simulink model "clothoidSequenceSimulation"  (R2022a)
settings: Solver=ode45  StartTime=0.0  StopTime=S  MaxStep=.1  RelTol=1e-3  EnableMultiTasking=on
values from neighbouring files (symbols this model uses):
  theta0 = 5/180*pi    (= 0.0872664625997)    [errorConnection_v1.m]    (also in errorConnection_v2.m; errorConnection_v3.m = 0.174532925199)
  y0 = 0.5    [errorConnection_v2.m]    (also in errorConnection_v3.m = 0)
settings Model: Creator=klaus  LastModifiedBy=schmidt
settings SolverCC: AlgebraicLoopSolver=TrustRegion
settings DataIOCC: LimitDataPoints=on  SaveFormat=Array  ReturnWorkspaceOutputs=off
settings OptimizationCC: LifeSpan=inf
settings DebuggingCC: UnderspecifiedInitializationDetection=Classic  MergeDetectMultiDrivingBlocksExec=none  SolverPrmCheckMsg=warning  UnconnectedInputMsg=warning  UnconnectedOutputMsg=warning  UnconnectedLineMsg=warning  StateNameClashWarn=warning  SFUnexpectedBacktrackingDiag=warning  SFNoUnconditionalDefaultTransitionDiag=warning  SFExecutionAtInitializationDiag=none  SFMachineParentedDataDiag=warning  ArithmeticOperatorsInVariantConditions=warning
settings HardwareCC: ProdBitPerPointer=32  ProdBitPerSizeT=32  ProdBitPerPtrDiffT=32  ProdLargestAtomicFloat=None  ProdIntDivRoundTo=Undefined  ProdEndianess=Unspecified  ProdWordSize=32  ProdHWDeviceType=32-bit Generic
settings ModelReferenceCC: PropagateSignalLabelsOutOfModel=off
settings SFSimCC: SimUseLocalCustomCode=off  CustomCodeUndefinedFunction=UseInterfaceOnly
settings RTWCC: RTWUseLocalCustomCode=off
settings CodeAppCC: StateflowObjectComments=on
settings GRTTargetCC: TargetLangStandard=C89/C90 (ANSI)
settings ConfigComp: CovMetricSettings=dw  CovSaveCumulativeToWorkspaceVar=on  CovSaveSingleToWorkspaceVar=on  CovExternalEMLEnable=off

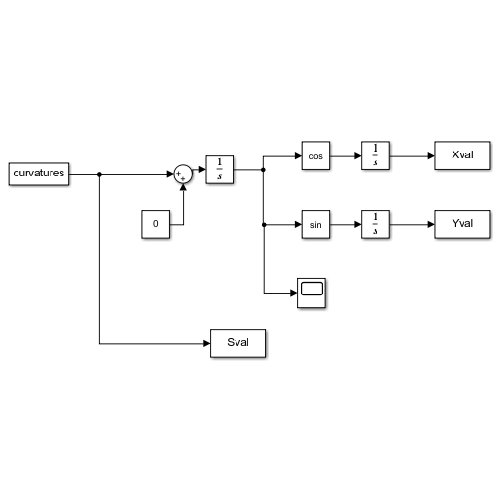
[thumbnail: Simulink's stored preview of the top-level diagram]
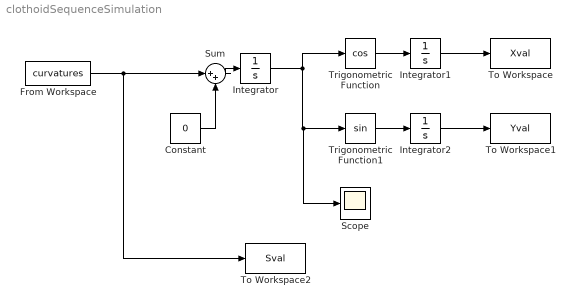
== system clothoidSequenceSimulation ==
  Constant : Constant  Value=0
  From Workspace : FromWorkspace  VariableName=curvatures
  Integrator : Integrator  InitialCondition=theta0
  Integrator1 : Integrator
  Integrator2 : Integrator  InitialCondition=y0
  Scope : Scope
  Sum : Sum  Inputs=|++
  To Workspace : ToWorkspace  VariableName=Xval  SampleTime=-1
  To Workspace1 : ToWorkspace  VariableName=Yval  SampleTime=-1
  To Workspace2 : ToWorkspace  VariableName=Sval  SampleTime=-1
  Trigonometric Function : Trigonometry  Operator=cos
  Trigonometric Function1 : Trigonometry
  wires:
  Integrator/1 -> Scope/1, Trigonometric Function1/1, Trigonometric Function/1
  Trigonometric Function/1 -> Integrator1/1
  Trigonometric Function1/1 -> Integrator2/1
  Integrator1/1 -> To Workspace/1
  Integrator2/1 -> To Workspace1/1
  Sum/1 -> Integrator/1
  From Workspace/1 -> Sum/1, To Workspace2/1
  Constant/1 -> Sum/2
